simulink model "PEMFuelCellSystem_Cathode_cEGR_ExternalMembraneHumidifier_v01"  (R2025b)
settings: Solver=VariableStepAuto  StartTime=0.0  StopTime=100  MaxStep=0.1  RelTol=1e-3  AbsTol=1e-3
model workspace (MAT data in the model file):
  Gas_properties_block = 'PEMFuelCellSystem_Before_v01/Anode_Hydrogen_BOP/Gas Mixture
Properties'
  Gas_properties_candidates{1} = 'PEMFuelCellSystem_Before_v01/Anode_Hydrogen_BOP/Gas Mixture
    | Properties'
  T_TLU = [223.15 228.15 233.15 238.15 243.15 248.15 253.15 258.15 263.15 268.15 272.66 273.15 273.66 278.15 283.15 288.15 293.15 298.15 303.15 308.15 313.15 318.15 323.15 328.15 333.15 338.15 343.15 348.15 353.15 358.15 363.15 368.15 373.15 378.15 383.15 388.15 393.15 398.15 403.15 408.15 413.15 418.15 423.15 428.15 433.15 438.15 443.15 448.15 453.15 458.15 463.15 468.15 473.15 478.15 483.15 488.15 493.15 498.15 503.15 508.15 513.15 518.15 523.15 528.15 533.15 538.15 543.15 548.15 553.15 558.15 563.15 568.15 573.15 578.15 583.15 588.15 593.15 598.15 603.15 608.15 613.15 618.15 623.15 628.15 633.15 638.15 643.15 646.596 647.596 648.15 653.15 658.15 663.15 668.15 673.15 678.15 683.15 688.15 693.15 698.15 703.15 708.15 713.15 718.15 723.15 728.15 733.15 738.15 743.15 748.15 753.15 758.15 763.15 768.15 773.15]
  air_control_min_current_A = 3.8
  anode_separator_D = 0.02
  anode_separator_T0 = 20
  anode_separator_area = 0.000314159265359
  anode_separator_dp_nominal = 0.0005
  anode_separator_extra_length = 0.04
  anode_separator_laminar_fraction = 0.001
  anode_separator_length = 0.12
  anode_separator_mdot_nominal = 0.01
  anode_separator_p0 = 0.101325
  anode_separator_roughness = 1.5e-05
  anode_tube_D = 0.02
  cathode_channel_dp_nominal_MPa = 0.0368422
  cathode_channel_flow_area_m2 = 0.00403764556423
  cathode_channel_laminar_fraction = 0.5
  cathode_channel_mdot_nominal_kg_s = 0.27182
  cathode_outlet_chamber_V = 0.2
  cathode_separator_D = 0.05
  cathode_separator_T0 = 20
  cathode_separator_area = 0.00407150407905
  cathode_separator_dp_nominal = 0.002
  cathode_separator_extra_length = 0.05
  cathode_separator_laminar_fraction = 0.001
  cathode_separator_length = 0.15
  cathode_separator_mdot_nominal = 0.40798
  cathode_separator_p0 = 0.101325
  cathode_separator_roughness = 1.5e-05
  cathode_tube_D = 0.05
  cegr_comp_map_t_denom_epsilon = 1e-09
  cegr_cond_tau = 1
  cegr_inlet_mixer_p0 = 0.101325
  cegr_outlet_chamber_p0 = 0.101325
  cegr_pipe_D = 0.072
  cegr_pipe_area = 0.00407150407905
  cegr_pipe_extra_length = 0.1
  cegr_pipe_length = 0.5
  cegr_pipe_p0 = 0.101325
  cegr_pipe_roughness = 1.5e-05
  cegr_valve_max_area = 0.001
  cegr_valve_open_min_area = 1e-10
  comp_inlet_mixer_V = 0.1
  comp_mdot_corr_TLU = [0  0.28  0.56; 0  0.26  0.52; 0  0.24  0.48; 0  0.22  0.44; 0  0.2  0.4]
  comp_p_ratio_TLU = [1 1.5 2 2.5 3]
  comp_rpm_TLU = [0 50000 80000]
  coolant_num_layers = 20
  coolant_num_passes = 12
  coolant_tube_D = 0.05
  coolant_w_channels = 1
  drive_cycle_current = [0 0 100 100]
  drive_cycle_power = [0 0 40 40]
  drive_cycle_time = [0 0.5 60.5 600]
  drive_cycle_voltage = [427.6 427.6 410 410]
  env_RH = 0.5
  env_T = 20
  env_p = 0.101325
  env_pSat_H2O = 0.00233931818334
  env_yH20 = 0.0115436377169
  env_yO2 = 0.21
  exhaust_bp_valve_control_Ki_area_per_MPa_s = 0.002
  exhaust_bp_valve_max_area = 0.00134
  exhaust_bp_valve_open_min_area = 1e-10
  focused_anode_boundary_T_C = 20
  focused_anode_feed_p_MPa_abs = 0.3
  focused_anode_inlet_mdot_kg_s = 0.008
  focused_anode_inlet_p_MPa_abs = 0.161325
  focused_anode_outlet_p_MPa_abs = 0.101325
  focused_anode_pipe_area = 0.00246300864041
  focused_anode_pipe_extra_length = 0.1
  focused_anode_pipe_length = 1
  focused_anode_pipe_roughness = 1.5e-05
  focused_anode_yH2 = 0.9997
  focused_cathode_inlet_temperature_C = 58.9
  focused_stack_temperature_C = 80
  humidifier_bypass_mode = "command_gain"
  intercooler_Dh = 0.05
  intercooler_T0 = 20
  intercooler_area = 0.00785398163397
  intercooler_cond_tau = 1
  intercooler_dp_nominal = 0.005
  intercooler_extra_length = 0.05
  intercooler_laminar_fraction = 0.001
  intercooler_length = 0.25
  intercooler_mdot_nominal = 0.40798
  intercooler_p0 = 0.101325
  intercooler_roughness = 1.5e-05
  membrane_humidifier_dry_area_m2 = 0.01
  membrane_humidifier_dry_extra_length_m = 0.1
  membrane_humidifier_dry_hydraulic_diameter_m = 0.05
  membrane_humidifier_dry_length_m = 1
  membrane_humidifier_dry_roughness_m = 1.5e-05
  membrane_humidifier_heat_conductivity_W_per_m_K = 5
  membrane_humidifier_temperature_transfer_time_constant_s = 0.2
  membrane_humidifier_water_transfer_conductance_kg_s_Pa = 1e-08
  membrane_humidifier_water_transfer_time_constant_s = 0.5
  membrane_humidifier_wet_area_m2 = 0.01
  membrane_humidifier_wet_extra_length_m = 0.1
  membrane_humidifier_wet_hydraulic_diameter_m = 0.05
  membrane_humidifier_wet_length_m = 1
  membrane_humidifier_wet_roughness_m = 1.5e-05
  pSat_H2O_TLU = [0.0039376926592 0.00720321689378 0.0128411282011 0.0223441068076 0.0380050105363 0.0632733889962 0.103238678713 0.165273175188 0.259872929049 0.401739659013 0.586936061043 0.611151401419 0.634239116603 0.872575113841 1.22819893069 1.70579291606 2.33931818334 3.16992933887 4.24697083683 5.62901610671 7.38493807375 9.59499884361 12.3519458375 15.7621015462 19.9464343078 25.0415980794 31.2009300265 38.5953958474 47.4144740302 57.866971652 70.1817658151 84.6084663194 101.41799666 120.903091855 143.378712949 169.182379251 198.67442048 232.238151946 270.279976785 313.229419961 361.5390994 415.684640163 476.16453797 543.499978781 618.234621425 700.934350503 792.187006981 892.602104065 1002.81053608 1123.46428821 1255.23615516 1398.81947697 1554.92790047 1724.29517523 1907.67499353 2105.84088402 2319.5861702 2549.72400533 2797.08749693 3062.5299355 3346.92514427 3651.16796903 3976.17493065 4322.88506654 4692.2609923 5085.29022074 5502.98678301 5946.3932056 6416.58290953 6914.66311353 7441.77834442 7999.11468638 8587.90494083 9209.43492415 9865.05121118 10556.1707482 11284.2929275 12051.0149487 12858.0516 13707.2609154 14600.6773719 15540.5540963 16529.415139 17570.1228342 18666.0066449 19821.3641683 21043.5631475 21931.4055737 22037.430306 22037.431306 22037.432306 22037.433306 22037.434306 22037.435306 22037.436306 22037.437306 22037.438306 22037.439306 22037.440306 22037.441306 22037.442306 22037.443306 22037.444306 22037.445306 22037.446306 22037.447306 22037.448306 22037.449306 22037.450306 22037.451306 22037.452306 22037.453306 22037.454306 22037.455306 22037.456306]
  pSat_TLU = [3379.45709837  3379.45809837  3379.45909837  3379.46009837  3379.46109837  3379.46209837  3379.46309837  3379.46409837  3379.46509837  3379.46609837  3379.46709837  3379.46809837  3379.46909837  3379.47009837  3379.47109837  3379.47209837  3379.47309837  3379.47409837  3379.47509837  3379.47609837  3379.47709837  3379.47809837  3379.47909837  3379.48009837  3379.48109837  3379.48209837  3379.48309837  3379.48409837  3379.48509837  3379.48609837  3379.48709837  3379.48809837  3379.48909837  3379.49009837  3379.49109837  3379.49209837  3379.49309837  3379.49409837  3379.49509837  3379.49609837  3379.49709837  3379.49809837  3379.49909837  3379.50009837  3379.50109837  3379.50209837  3379.50309837  3379.50409837  3379.50509837  3379.50609837  3379.50709837  3379.50809837  3379.50909837  3379.51009837  3379.51109837  3379.51209837  3379.51309837  3379.51409837  3379.51509837  3379.51609837  3379.51709837  3379.51809837  3379.51909837  3379.52009837  3379.52109837  3379.52209837  3379.52309837  3379.52409837  3379.52509837  3379.52609837  3379.52709837  3379.52809837  3379.52909837  3379.53009837  3379.53109837  3379.53209837  3379.53309837  3379.53409837  3379.53509837  3379.53609837  3379.53709837  3379.53809837  3379.53909837  3379.54009837  3379.54109837  3379.54209837  3379.54309837  3379.54409837  3379.54509837  3379.54609837  3379.54709837  3379.54809837  3379.54909837  3379.55009837  3379.55109837  3379.55209837  3379.55309837  3379.55409837  3379.55509837  3379.55609837  3379.55709837  3379.55809837  3379.55909837  3379.56009837  3379.56109837  3379.56209837  3379.56309837  3379.56409837  3379.56509837  3379.56609837  3379.56709837  3379.56809837  3379.56909837  3379.57009837  3379.57109837; 5023.40410987  5023.40510987  5023.40610987  5023.40710987  5023.40810987  5023.40910987  5023.41010987  5023.41110987  5023.41210987  5023.41310987  5023.41410987  5023.41510987  5023.41610987  5023.41710987  5023.41810987  5023.41910987  5023.42010987  5023.42110987  5023.42210987  5023.42310987  5023.42410987  5023.42510987  5023.42610987  5023.42710987  5023.42810987  5023.42910987  5023.43010987  5023.43110987  5023.43210987  5023.43310987  5023.43410987  5023.43510987  5023.43610987  5023.43710987  5023.43810987  5023.43910987  5023.44010987  5023.44110987  5023.44210987  5023.44310987  5023.44410987  5023.44510987  5023.44610987  5023.44710987  5023.44810987  5023.44910987  5023.45010987  5023.45110987  5023.45210987  5023.45310987  5023.45410987  5023.45510987  5023.45610987  5023.45710987  5023.45810987  5023.45910987  5023.46010987  5023.46110987  5023.46210987  5023.46310987  5023.46410987  5023.46510987  5023.46610987  5023.46710987  5023.46810987  5023.46910987  5023.47010987  5023.47110987  5023.47210987  5023.47310987  5023.47410987  5023.47510987  5023.47610987  5023.47710987  5023.47810987  5023.47910987  5023.48010987  5023.48110987  5023.48210987  5023.48310987  5023.48410987  5023.48510987  5023.48610987  5023.48710987  5023.48810987  5023.48910987  5023.49010987  5023.49110987  5023.49210987  5023.49310987  5023.49410987  5023.49510987  5023.49610987  5023.49710987  5023.49810987  5023.49910987  5023.50010987  5023.50110987  5023.50210987  5023.50310987  5023.50410987  5023.50510987  5023.50610987  5023.50710987  5023.50810987  5023.50910987  5023.51010987  5023.51110987  5023.51210987  5023.51310987  5023.51410987  5023.51510987  5023.51610987  5023.51710987  5023.51810987; 1277.63968517  1277.64068517  1277.64168517  1277.64268517  1277.64368517  1277.64468517  1277.64568517  1277.64668517  1277.64768517  1277.64868517  1277.64968517  1277.65068517  1277.65168517  1277.65268517  1277.65368517  1277.65468517  1277.65568517  1277.65668517  1277.65768517  1277.65868517  1277.65968517  1277.66068517  1277.66168517  1277.66268517  1277.66368517  1277.66468517  1277.66568517  1277.66668517  1277.66768517  1277.66868517  1277.66968517  1277.67068517  1277.67168517  1277.67268517  1277.67368517  1277.67468517 ...(+2889 chars)]
  radiator_H = 0.5
  radiator_L = 1
  radiator_N_fins = 12000
  radiator_N_tubes = 25
  radiator_W = 0.025
  radiator_air_area_fins = 11.5625
  radiator_air_area_primary = 1.223125
  radiator_cp = 910
  radiator_eta_fin = 0.7
  radiator_fin_spacing = 0.002
  radiator_gap_H = 0.0192708333333
  radiator_rho = 2700
  radiator_t_wall = 0.0001
  radiator_tube_H = 0.0015
  radiator_tube_Leq = 2.5
  routeA_air_control_mode_id = 2
  routeA_air_pid_Ki = 0.5
  routeA_air_pid_Kp = 5
  routeA_anode_inlet_pressure_MPa_abs = 0.161325
  routeA_anode_purge_enable = 1
  routeA_anode_purge_off_n2_mole_fraction = 0.1
  routeA_anode_purge_on_n2_mole_fraction = 0.5
  routeA_anode_recirculation_base_command = 0.2
  routeA_anode_recirculation_current_gain_A_inv = 0.00204081632653
  routeA_anode_rh_setpoint = 1
  routeA_backpressure_control_mode_id = 1
  routeA_cathode_humidifier_gain = 1
  routeA_cathode_rh_setpoint = 1
  routeA_cegr_enabled = 1
  routeA_cegr_valve_mode_id = 1
  routeA_command_profile = [0  0.101325  20  0.21  0.0115436377169  0.045  3  0.5  0.161325  1  1  0  70  20  0.9997  0.161325  1  0.2  0.00204081632653  1  0.5  0.1  80; 0.5  0.101325  20  0.21  0.0115436377169  0.045  3  0.5  0.161325  1  1  0  70  20  0.9997  0.161325  1  0.2  0.00204081632653  1  0.5  0.1  80; 60.5  0.101325  20  0.21  0.0115436377169  0.045  3  0.5  0.161325  1  1  0.1  70  20  0.9997  0.161325  1  0.2  0.00204081632653  1  0.5  0.1  80; 600  0.101325  20  0.21  0.0115436377169  0.045  3  0.5  0.161325  1  1  0.1  70  20  0.9997  0.161325  1  0.2  0.00204081632653  1  0.5  0.1  80]
  routeA_command_profile_baseline = [0.101325 20 0.21 0.0115436377169 0.045 3 0.5 0.1613 1 1 0 70 20 0.9997 0.161325 1 0.2 0.00204081632653 1 0.5 0.1 80]
  routeA_command_profile_fields = ["cathode_source_pressure_MPa_abs" "cathode_source_temperature_C" "cathode_source_o2_mole_fraction" "cathode_source_h2o_mole_fraction" "air_target_mdot_kg_s" "air_target_oer" "air_direct_command" "cathode_outlet_pressure_MPa_abs" "cathode_humidifier_rh" "cathode_humidifier_gain" "cegr_ratio" "anode_source_pressure_MPa_abs" "anode_source_temperature_C" "anode_source_h2_mole_fraction" "anode_inlet_pressure_MPa_abs" "anode_humidifier_rh" "anode_recirculation_base" "anode_recirculation_current_gain_A_inv" "anode_purge_enable" "anode_purge_on_n2_mole_fraction" "anode_purge_off_n2_mole_fraction" "stack_temperature_set_C"]
  routeA_command_profile_schema = "RouteA_Command_Profile_v10"
  routeA_current_default_ref_A = 28
  routeA_egr_control_Ki_area = 3.92699081699e-05
  routeA_egr_control_Kp_area = 0.000196349540849
  routeA_egr_control_mode_id = 1
  routeA_egr_target_input_mode_id = 1
  routeA_egr_valve_actuator_tau = 0.5
  routeA_egr_valve_area_direct = 3.92699081699e-06
  routeA_external_case_enabled = 0
  routeA_parameter_layer = "platform_default"
  routeA_stack_temperature_set_C = 80
  routeA_target_egr_ratio_comp_in = 0.02
  routeA_voltage_current_max_A = 392
  routeA_voltage_current_min_A = 0
  routeA_voltage_default_ref_V = 394.9
  routeA_voltage_pi_Ki = 0.05
  routeA_voltage_pi_Kp = 1
  separator_condensation_enabled = 1
  separator_l2_efficiency = 0.5
  separator_l2_source = "l2_saturation_excess_estimator"
  stack_alpha = 1
  stack_area = 380
  stack_iL = 2.5
  stack_io = 2e-14
  stack_mea_cp = 870
  stack_mea_rho = 1800
  stack_num_cells = 606
  stack_num_channels = 8
  stack_t_gdl = 250
  stack_t_membrane = 125
  stack_w_channels = 1.16496474502
  tank_T = 20
  tank_V = 120
  tank_p = 70
  tank_yH2 = 0.9997
libraries: nesl_utility x57, FuelCell_lib x39, fl_lib x24, slpidlib x4
(part 1 of 6)
settings Model: Creator=ADMIN  LastModifiedBy=ADMIN
settings SolverCC: AutoScaleAbsTol=off  MaxConsecutiveMinStep=10  AlgebraicLoopSolver=TrustRegion  MaxZcPerStep=1.0
settings DataIOCC: SaveFormat=Array  ReturnWorkspaceOutputs=off
settings DebuggingCC: UnconnectedInputMsg=warning  UnconnectedOutputMsg=warning  UnconnectedLineMsg=warning  SymbolicDimsDataTypeCodeGenerationDiagnostic=none
settings ModelReferenceCC: EnableRefExpFcnMdlSchedulingChecks=on
settings SFSimCC: CustomCodeUndefinedFunction=UseInterfaceOnly
settings RTWCC: GPUComputeCapability=3.5  DLArmComputeVersion=19.05
settings SimscapeCC: SimscapeLogType=all  SimscapeLogSimulationStatistics=on  SimscapeLogName=simlog_PEMFuelCellSystem_GasMixture_cEGR_RouteA_v01  SimscapeLogDataHistory=20000.0

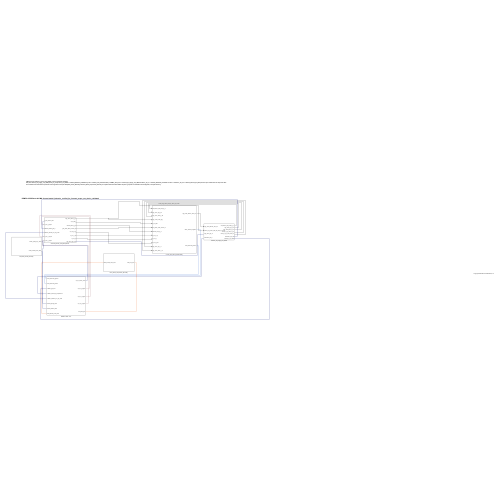
[thumbnail: Simulink's stored preview of the top-level diagram]
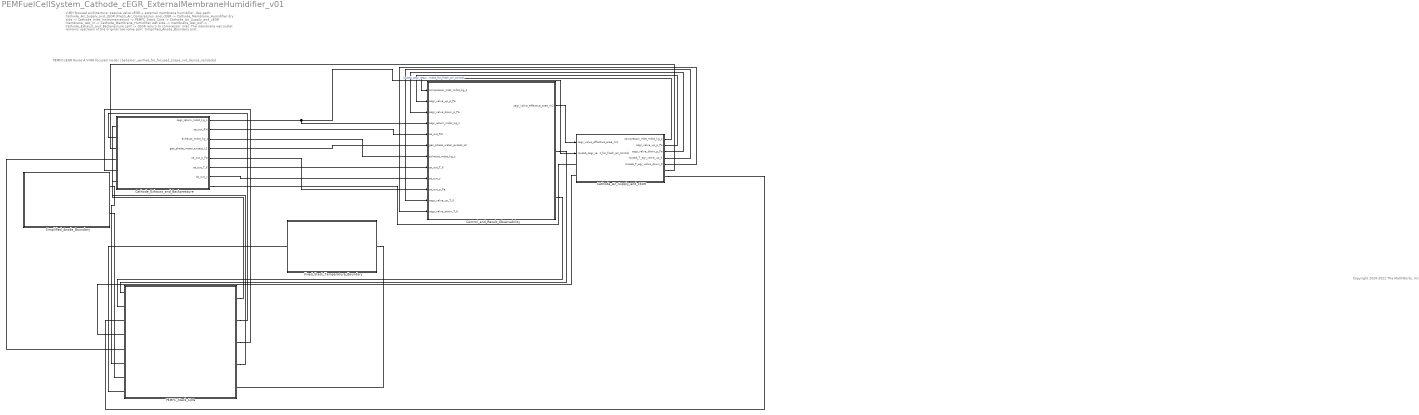
== system PEMFuelCellSystem_Cathode_cEGR_ExternalMembraneHumidifier_v01 ==
  note: PEMFC-cEGR Route A V-MH focused model | behavior_verified_for_focused_scope_not_device_validated
  note: V-MH focused architecture: passive valve cEGR + external membrane humidifier.
      | Gas path: Cathode_Air_Supply_and_cEGR [Fresh_Air_Compression_and_cEGR -> Cathode_Membrane_Humidifier dry side -> Cathode_Inlet_Instrumentation] -> PEMFC_Stack_Core -> Cathode_Air_Supply_and_cEGR membrane_wet_in -> Cathode_Membrane_Humidifier wet side -> membrane_wet_out -> Cathode_Exhaust_and_Backpressure split -> cEGR return to compressor inlet.
      | The membrane wet outlet remains upstream of the original two-valve split. Simplified_Anode_Boundary and Fixed_Stack_Temperature_Boundary are explicit model boundaries. Water output is a gas-phase L2 saturation-excess diagnostic, not liquid inventory.
  note: Copyright 2020-2022 The MathWorks, Inc.
  Cathode_Air_Supply_and_cEGR : Subsystem
  Cathode_Exhaust_and_Backpressure : Subsystem  Description=Common backpressure, gas-phase boundary, return/exhaust split and cathode-outlet result observation.
  Control_and_Result_Observability : Subsystem  Description=Electrical load, cathode/cEGR control, stack measurements and auditable result logging.
  Fixed_Stack_Temperature_Boundary : Subsystem  Description=Fixed stack temperature source and Simscape solver configuration. This is not a cooling-system model.
  PEMFC_Stack_Core : Subsystem  Description=MEA, anode/cathode gas channels, cathode outlet chamber and stack thermal mass.
  Simplified_Anode_Boundary : Subsystem  Description=Hydrogen mass-flow inlet, fixed feed/outlet reservoirs and minimal insulated outlet pipe. No anode humidifier, recirculation or purge BOP.
  wires:
  Cathode_Exhaust_and_Backpressure/6(ca_out_T_K) -> Control_and_Result_Observability/8(ca_out_T_K)
  Cathode_Exhaust_and_Backpressure/5(ca_out_p_Pa) -> Control_and_Result_Observability/10(ca_out_p_Pa)
  Cathode_Exhaust_and_Backpressure/3(exhaust_mdot_kg_s) -> Control_and_Result_Observability/7(exhaust_mdot_kg_s)
  Cathode_Exhaust_and_Backpressure/2(ca_out_RH) -> Control_and_Result_Observability/5(ca_out_RH)
  Cathode_Exhaust_and_Backpressure/1(cegr_return_mdot_kg_s) -> Cathode_Air_Supply_and_cEGR/2(routeA_cegr_return_mdot_for_fresh_air_control), Control_and_Result_Observability/4(cegr_return_mdot_kg_s)  "routeA_cegr_return_mdot_for_fresh_air_control"
  Cathode_Exhaust_and_Backpressure/7(ca_out_y) -> Control_and_Result_Observability/9(ca_out_y)
  Cathode_Exhaust_and_Backpressure/4(gas_phase_water_excess_L2) -> Control_and_Result_Observability/6(gas_phase_water_excess_L2)
  Control_and_Result_Observability/1(cegr_valve_effective_area_m2) -> Cathode_Air_Supply_and_cEGR/1(cegr_valve_effective_area_m2)
  Cathode_Air_Supply_and_cEGR/1(compressor_inlet_mdot_kg_s) -> Control_and_Result_Observability/1(compressor_inlet_mdot_kg_s)
  Cathode_Air_Supply_and_cEGR/2(cegr_valve_up_p_Pa) -> Control_and_Result_Observability/2(cegr_valve_up_p_Pa)
  Cathode_Air_Supply_and_cEGR/3(cegr_valve_down_p_Pa) -> Control_and_Result_Observability/3(cegr_valve_down_p_Pa)
  Cathode_Air_Supply_and_cEGR/4(routeA_T_egr_valve_up_K) -> Control_and_Result_Observability/11(cegr_valve_up_T_K)
  Cathode_Air_Supply_and_cEGR/5(routeA_T_egr_valve_down_K) -> Control_and_Result_Observability/12(cegr_valve_down_T_K)
  connections:
  Control_and_Result_Observability/RConn2 -- PEMFC_Stack_Core/LConn2
  Control_and_Result_Observability/RConn1 -- PEMFC_Stack_Core/LConn1
  Simplified_Anode_Boundary/RConn2 -- PEMFC_Stack_Core/LConn7
  Simplified_Anode_Boundary/RConn1 -- PEMFC_Stack_Core/LConn6
  PEMFC_Stack_Core/RConn2 -- Cathode_Exhaust_and_Backpressure/LConn2
  PEMFC_Stack_Core/RConn4 -- Cathode_Exhaust_and_Backpressure/LConn6
  PEMFC_Stack_Core/LConn5 -- Cathode_Exhaust_and_Backpressure/LConn4
  PEMFC_Stack_Core/RConn1 -- Cathode_Exhaust_and_Backpressure/LConn1
  PEMFC_Stack_Core/RConn3 -- Cathode_Exhaust_and_Backpressure/LConn5
  Fixed_Stack_Temperature_Boundary/LConn1 -- PEMFC_Stack_Core/LConn8
  Fixed_Stack_Temperature_Boundary/RConn1 -- PEMFC_Stack_Core/RConn5
  Cathode_Air_Supply_and_cEGR/RConn1 -- Cathode_Exhaust_and_Backpressure/LConn3
  Cathode_Exhaust_and_Backpressure/RConn1 -- Cathode_Air_Supply_and_cEGR/LConn1
  Cathode_Air_Supply_and_cEGR/RConn2 -- PEMFC_Stack_Core/LConn3
  PEMFC_Stack_Core/LConn4 -- Cathode_Air_Supply_and_cEGR/LConn2

== system PEMFuelCellSystem_Cathode_cEGR_ExternalMembraneHumidifier_v01/Cathode_Air_Supply_and_cEGR ==
  cegr_valve_effective_area_m2 : Inport
  routeA_cegr_return_mdot_for_fresh_air_control : Inport  Port=2
  Cathode_Inlet_Instrumentation : Subsystem  Description=In-line cathode inlet sensors and V-SH RH/species mass-flow recording.
  Cathode_Membrane_Humidifier : Subsystem  Description=V-MH membrane humidifier shell: two official Pipe (FC) gas volumes, equal/opposite H2O MIn/TIn interface, and conservative wall heat transfer. Cross-membrane transfer is added in the next staged step.
  Fresh_Air_Compression_and_cEGR : Subsystem  Description=Function: fresh-air compression/intercooling, compressor-inlet cEGR mixing, passive return valve and insulated return pipe. Input: valve effective area. Outputs: compressor-inlet mass flow plus valve upstream/downstream pressure and temperature. The return-pipe side species source is explicitly zero because V-SH contains no external reaction or separator in this pipe.
  membrane_wet_out : PMIOPort  Side=Right
  cegr_return_gas_in : PMIOPort  Port=2  Side=Left
  cathode_air_to_stack : PMIOPort  Port=3  Side=Right
  membrane_wet_in : PMIOPort  Port=4  Side=Left
  compressor_inlet_mdot_kg_s : Outport
  cegr_valve_up_p_Pa : Outport  Port=2
  cegr_valve_down_p_Pa : Outport  Port=3
  routeA_T_egr_valve_up_K : Outport  Port=4
  routeA_T_egr_valve_down_K : Outport  Port=5
  wires:
  Fresh_Air_Compression_and_cEGR/4(cegr_valve_up_T_K) -> routeA_T_egr_valve_up_K/1  "routeA_T_egr_valve_up_K"
  Fresh_Air_Compression_and_cEGR/2(cegr_valve_up_p_Pa) -> cegr_valve_up_p_Pa/1
  Fresh_Air_Compression_and_cEGR/1(compressor_inlet_mdot_kg_s) -> compressor_inlet_mdot_kg_s/1
  Fresh_Air_Compression_and_cEGR/3(cegr_valve_down_p_Pa) -> cegr_valve_down_p_Pa/1
  Fresh_Air_Compression_and_cEGR/5(cegr_valve_down_T_K) -> routeA_T_egr_valve_down_K/1  "routeA_T_egr_valve_down_K"
  cegr_valve_effective_area_m2/1 -> Fresh_Air_Compression_and_cEGR/1(cegr_valve_effective_area_m2)
  routeA_cegr_return_mdot_for_fresh_air_control/1 -> Fresh_Air_Compression_and_cEGR/2(cegr_return_mdot_kg_s)
  connections:
  Cathode_Membrane_Humidifier/RConn1 -- Cathode_Inlet_Instrumentation/LConn1
  Fresh_Air_Compression_and_cEGR/RConn1 -- Cathode_Membrane_Humidifier/LConn1
  cegr_return_gas_in/RConn1 -- Fresh_Air_Compression_and_cEGR/LConn1
  Cathode_Membrane_Humidifier/RConn2 -- membrane_wet_out/RConn1
  Cathode_Inlet_Instrumentation/RConn1 -- cathode_air_to_stack/RConn1
  membrane_wet_in/RConn1 -- Cathode_Membrane_Humidifier/LConn2

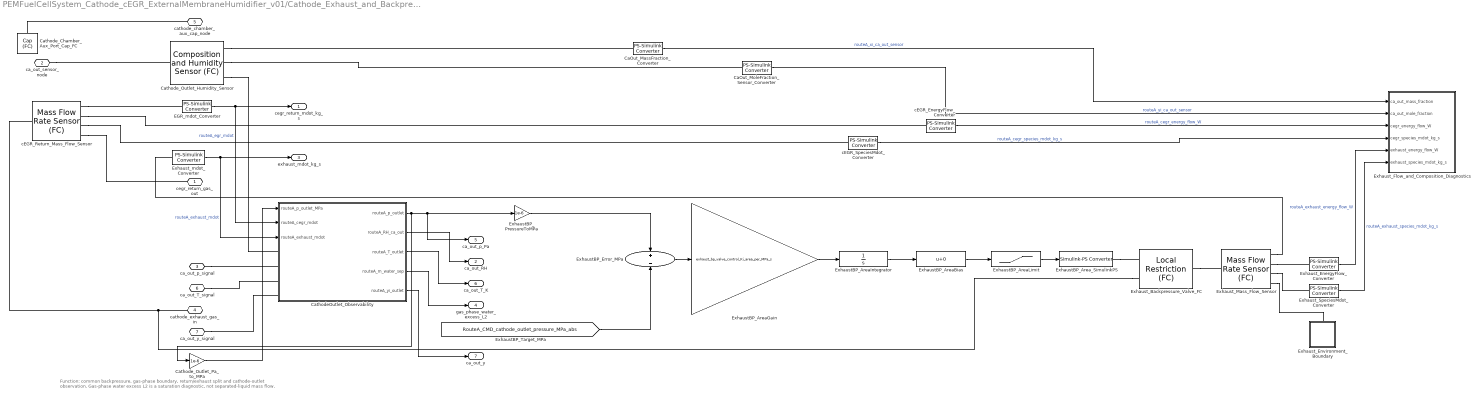
== system PEMFuelCellSystem_Cathode_cEGR_ExternalMembraneHumidifier_v01/Cathode_Exhaust_and_Backpressure ==
  note: Function: common backpressure, gas-phase boundary, return/exhaust split and cathode-outlet observation.
      | Gas-phase water excess L2 is a saturation diagnostic, not separated-liquid mass flow.
  CaOut_MassFraction_Converter : nesl_utility/PS-Simulink Converter  Description=Convert cathode-outlet sensor mass fractions to a named diagnostic signal.  PhysicalDomain=network_engine_domain  SubClassName=ps_output  LeftPortType=input  RightPortType=output  PseudoPeriodic=off  Frequencies=[]  VectorFormat=inherit  Unit=1  AffineConversion=off
  CaOut_MoleFraction_Sensor_Converter : nesl_utility/PS-Simulink Converter  Description=Convert cathode-outlet sensor mole fractions to a named diagnostic signal; this is independent readback of the outlet state.  PhysicalDomain=network_engine_domain  SubClassName=ps_output  LeftPortType=input  RightPortType=output  PseudoPeriodic=off  Frequencies=[]  VectorFormat=inherit  Unit=1  AffineConversion=off
  CathodeOutlet_Observability : Subsystem  Description=Converts cathode-outlet physical signals and branch mass flows into V-SH result observables. Water output is a gas-phase L2 saturation-excess diagnostic, not separated liquid-water inventory.
  Cathode_Chamber_Aux_Port_Cap_FC : FuelCell_lib/elements/Cap (FC)  p_specify=off  p_priority=None  p=101325 Pa  p_nominal_specify=off  p_nominal_value=1  p_nominal_unit=Pa  x_i_specify=off  x_i_priority=None  x_i=[1; 0; 0; 0]  x_i_nominal_specify=off  x_i_nominal_value=1  x_i_nominal_unit=1  T_specify=off  T_priority=None  T=293.15 K  T_nominal_specify=off  T_nominal_value=1  T_nominal_unit=K
      settings: InternalSimscapePortConfiguration="{\"Bottom\":[],\"Left\":[{\"id\":\"A\",\"label\":\"A\",\"type\":\"FuelCell.FuelCell\"}],\"Right\":[],\"Top\":[]}"
  Cathode_Outlet_Humidity_Sensor : FuelCell_lib/sensors/Composition and Humidity Sensor (FC)
      settings: InternalSimscapePortConfiguration="{\"Bottom\":[],\"Left\":[{\"id\":\"A\",\"label\":\"A\",\"type\":\"FuelCell.FuelCell\"}],\"Right\":[{\"id\":\"x_i\",\"label\":\"x_i\",\"type\":\"output\"},{\"id\":\"y_i\",\"label\":\"y_i\",\"type\":\"output\"},{\"id\":\"W\",\"label\":\"W\",\"type\":\"output\"}],\"Top\":[]}"
  Cathode_Outlet_Pa_to_MPa : Gain  Gain=1e-6
  EGR_mdot_Converter : nesl_utility/PS-Simulink Converter  PhysicalDomain=network_engine_domain  SubClassName=ps_output  LeftPortType=input  RightPortType=output  PseudoPeriodic=off  Frequencies=[]  VectorFormat=inherit  Unit=inherit  AffineConversion=off
  ExhaustBP_AreaBias : Bias
  ExhaustBP_AreaGain : Gain  Gain=exhaust_bp_valve_control_Ki_area_per_MPa_s
  ExhaustBP_AreaIntegrator : Integrator  InitialCondition=0.5*exhaust_bp_valve_max_area  LimitOutput=on  UpperSaturationLimit=exhaust_bp_valve_max_area  LowerSaturationLimit=exhaust_bp_valve_open_min_area
  ExhaustBP_AreaLimit : Saturate  UpperLimit=exhaust_bp_valve_max_area  LowerLimit=exhaust_bp_valve_open_min_area
  ExhaustBP_Area_SimulinkPS : nesl_utility/Simulink-PS Converter  PhysicalDomain=network_engine_domain  SubClassName=ps_input  LeftPortType=input  RightPortType=output  PseudoPeriodic=off  Frequencies=[]  NoiseDistribution=none  NoiseParameters=[]  Unit=m^2  AffineConversion=off  FilteringAndDerivatives=provide  SimscapeFilterOrder=1  InputFilterTimeConstant=0.001  UdotUserProvided=0
  ExhaustBP_Error_MPa : Sum  Inputs=+-
  ExhaustBP_PressureToMPa : Gain  Gain=1e-6
  Exhaust_Backpressure_Valve_FC : FuelCell_lib/elements/Local Restriction (FC)  const_area=false  restriction_area=exhaust_bp_valve_open_min_area m^2  min_area=exhaust_bp_valve_open_min_area m^2  max_area=exhaust_bp_valve_max_area m^2  area=0.01 m^2  Cd=0.64  B_lam=0.999
      settings: InternalSimscapePortConfiguration="{\"Bottom\":[],\"Left\":[{\"id\":\"AR\",\"label\":\"AR\",\"type\":\"input\"},{\"id\":\"A\",\"label\":\"A\",\"type\":\"FuelCell.FuelCell\"}],\"Right\":[{\"id\":\"B\",\"label\":\"B\",\"type\":\"FuelCell.FuelCell\"}],\"Top\":[]}"
  Exhaust_EnergyFlow_Converter : nesl_utility/PS-Simulink Converter  Description=Convert exhaust mixture energy flow [W] to a diagnostic signal. Positive direction is sensor A to B.  PhysicalDomain=network_engine_domain  SubClassName=ps_output  LeftPortType=input  RightPortType=output  PseudoPeriodic=off  Frequencies=[]  VectorFormat=inherit  Unit=W  AffineConversion=off
  Exhaust_Environment_Boundary : Subsystem  Tag=PublishSubsystem  Description=Cathode exhaust path to ambient. Applies the exhaust boundary after the common backpressure and gas-phase split.
      settings: PortSchema="{\"entries\":[{\"content\":{\"sides\":[{\"content\":{\"connectorIds\":[]},\"type\":\"ConnectorPlacement.EquallySpacedRectSide\",\"uuid\":\"6344d1cf-22ea-4a51-9588-07afca0fac15\"},{\"content\":{\"connectorIds\":[],\"side\":\"RIGHT\"},\"type\":\"ConnectorPlacement.EquallySpacedRectSide\",\"uuid\":\"a3908f81-9410-4056-87cd-9faba76d3fb8\"},{\"content\":{\"connectorIds\":[\"LConn1\"],\"side\":\"TOP\"},\"type\":\"ConnectorPlacement.EquallySpacedRectSide\",\"uuid\":\"a1c9e24d-adb9-4361-8e9b-feafccbbdb81\"}]},\"type\":\"ConnectorPlacement.EquallySpacedConnector\",\"uuid\":\"d5180d8f-18a0-491d-9fff-909db43c9aea\"}],\"packageUris\":[\"http://schema.mathworks.com/mf0/Connector/R2020b\"],\"version\":\"1.0\"}"
  Exhaust_Flow_and_Composition_Diagnostics : Subsystem  Description=Named observability consumer for cathode-outlet composition and cEGR/exhaust energy and species-flow diagnostics. These signals are measurements only and do not alter the gas network.
  Exhaust_Mass_Flow_Sensor : FuelCell_lib/sensors/Mass Flow Rate Sensor (FC)
      settings: InternalSimscapePortConfiguration="{\"Bottom\":[],\"Left\":[{\"id\":\"A\",\"label\":\"A\",\"type\":\"FuelCell.FuelCell\"}],\"Right\":[{\"id\":\"M\",\"label\":\"M\",\"type\":\"output\"},{\"id\":\"Phi_out\",\"label\":\"Phi\",\"type\":\"output\"},{\"id\":\"M_i\",\"label\":\"M_i\",\"type\":\"output\"},{\"id\":\"B\",\"label\":\"B\",\"type\":\"FuelCell.FuelCell\"}],\"Top\":[]}"
  Exhaust_SpeciesMdot_Converter : nesl_utility/PS-Simulink Converter  Description=Convert exhaust species mass-flow vector [kg/s] to a diagnostic signal. Positive direction is sensor A to B.  PhysicalDomain=network_engine_domain  SubClassName=ps_output  LeftPortType=input  RightPortType=output  PseudoPeriodic=off  Frequencies=[]  VectorFormat=inherit  Unit=kg/s  AffineConversion=off
  Exhaust_mdot_Converter : nesl_utility/PS-Simulink Converter  PhysicalDomain=network_engine_domain  SubClassName=ps_output  LeftPortType=input  RightPortType=output  PseudoPeriodic=off  Frequencies=[]  VectorFormat=inherit  Unit=inherit  AffineConversion=off
  cEGR_EnergyFlow_Converter : nesl_utility/PS-Simulink Converter  Description=Convert cEGR return mixture energy flow [W] to a diagnostic signal. Positive direction is sensor A to B.  PhysicalDomain=network_engine_domain  SubClassName=ps_output  LeftPortType=input  RightPortType=output  PseudoPeriodic=off  Frequencies=[]  VectorFormat=inherit  Unit=W  AffineConversion=off
  cEGR_Return_Mass_Flow_Sensor : FuelCell_lib/sensors/Mass Flow Rate Sensor (FC)
      settings: InternalSimscapePortConfiguration="{\"Bottom\":[],\"Left\":[{\"id\":\"A\",\"label\":\"A\",\"type\":\"FuelCell.FuelCell\"}],\"Right\":[{\"id\":\"M\",\"label\":\"M\",\"type\":\"output\"},{\"id\":\"Phi_out\",\"label\":\"Phi\",\"type\":\"output\"},{\"id\":\"M_i\",\"label\":\"M_i\",\"type\":\"output\"},{\"id\":\"B\",\"label\":\"B\",\"type\":\"FuelCell.FuelCell\"}],\"Top\":[]}"
  cEGR_SpeciesMdot_Converter : nesl_utility/PS-Simulink Converter  Description=Convert cEGR return species mass-flow vector [kg/s] to a diagnostic signal. Positive direction is sensor A to B.  PhysicalDomain=network_engine_domain  SubClassName=ps_output  LeftPortType=input  RightPortType=output  PseudoPeriodic=off  Frequencies=[]  VectorFormat=inherit  Unit=kg/s  AffineConversion=off
  cegr_return_gas_out : PMIOPort  Side=Right
  ca_out_sensor_node : PMIOPort  Port=2  Side=Left
  ca_out_p_signal : PMIOPort  Port=3  Side=Left
  cathode_exhaust_gas_in : PMIOPort  Port=4  Side=Left
  cathode_chamber_aux_cap_node : PMIOPort  Port=5  Side=Left
  ca_out_T_signal : PMIOPort  Port=6  Side=Left
  ca_out_y_signal : PMIOPort  Port=7  Side=Left
  cegr_return_mdot_kg_s : Outport
  ca_out_RH : Outport  Port=2
  exhaust_mdot_kg_s : Outport  Port=3
  gas_phase_water_excess_L2 : Outport  Port=4
  ca_out_p_Pa : Outport  Port=5
  ca_out_T_K : Outport  Port=6
  ca_out_y : Outport  Port=7
  wires:
  ExhaustBP_AreaIntegrator/1 -> ExhaustBP_AreaBias/1
  EGR_mdot_Converter/1 -> cegr_return_mdot_kg_s/1, CathodeOutlet_Observability/2(routeA_cegr_mdot)  "routeA_egr_mdot"
  Exhaust_mdot_Converter/1 -> exhaust_mdot_kg_s/1, CathodeOutlet_Observability/3(routeA_exhaust_mdot)  "routeA_exhaust_mdot"
  cEGR_EnergyFlow_Converter/1 -> Exhaust_Flow_and_Composition_Diagnostics/3(cegr_energy_flow_W)  "routeA_cegr_energy_flow_W"
  Cathode_Outlet_Pa_to_MPa/1 -> CathodeOutlet_Observability/1(routeA_p_outlet_MPa)
  CathodeOutlet_Observability/1(routeA_p_outlet) -> ca_out_p_Pa/1, ExhaustBP_PressureToMPa/1, Cathode_Outlet_Pa_to_MPa/1
  CathodeOutlet_Observability/2(routeA_RH_ca_out) -> ca_out_RH/1
  CaOut_MoleFraction_Sensor_Converter/1 -> Exhaust_Flow_and_Composition_Diagnostics/2(ca_out_mole_fraction)  "routeA_yi_ca_out_sensor"
  CathodeOutlet_Observability/3(routeA_T_outlet) -> ca_out_T_K/1
  CathodeOutlet_Observability/4(routeA_m_water_sep) -> gas_phase_water_excess_L2/1
  CathodeOutlet_Observability/5(routeA_yi_outlet) -> ca_out_y/1
  ExhaustBP_AreaGain/1 -> ExhaustBP_AreaIntegrator/1
  ExhaustBP_PressureToMPa/1 -> ExhaustBP_Error_MPa/1
  [RouteA_CMD_cathode_outlet_pressure_MPa_abs] -> ExhaustBP_Error_MPa/2
  CaOut_MassFraction_Converter/1 -> Exhaust_Flow_and_Composition_Diagnostics/1(ca_out_mass_fraction)  "routeA_xi_ca_out_sensor"
  ExhaustBP_AreaBias/1 -> ExhaustBP_AreaLimit/1
  ExhaustBP_Error_MPa/1 -> ExhaustBP_AreaGain/1
  cEGR_SpeciesMdot_Converter/1 -> Exhaust_Flow_and_Composition_Diagnostics/4(cegr_species_mdot_kg_s)  "routeA_cegr_species_mdot_kg_s"
  ExhaustBP_AreaLimit/1 -> ExhaustBP_Area_SimulinkPS/1
  Exhaust_EnergyFlow_Converter/1 -> Exhaust_Flow_and_Composition_Diagnostics/5(exhaust_energy_flow_W)  "routeA_exhaust_energy_flow_W"
  Exhaust_SpeciesMdot_Converter/1 -> Exhaust_Flow_and_Composition_Diagnostics/6(exhaust_species_mdot_kg_s)  "routeA_exhaust_species_mdot_kg_s"
  connections:
  Exhaust_Mass_Flow_Sensor/RConn3 -- Exhaust_SpeciesMdot_Converter/LConn1
  cEGR_Return_Mass_Flow_Sensor/RConn4 -- cegr_return_gas_out/RConn1
  Exhaust_Mass_Flow_Sensor/RConn1 -- Exhaust_mdot_Converter/LConn1
  cEGR_Return_Mass_Flow_Sensor/RConn2 -- cEGR_EnergyFlow_Converter/LConn1
  Cathode_Chamber_Aux_Port_Cap_FC/LConn1 -- cathode_chamber_aux_cap_node/RConn1
  Exhaust_Mass_Flow_Sensor/RConn2 -- Exhaust_EnergyFlow_Converter/LConn1
  ca_out_T_signal/RConn1 -- CathodeOutlet_Observability/LConn3
  cEGR_Return_Mass_Flow_Sensor/RConn3 -- cEGR_SpeciesMdot_Converter/LConn1
  cEGR_Return_Mass_Flow_Sensor/RConn1 -- EGR_mdot_Converter/LConn1
  ca_out_sensor_node/RConn1 -- Cathode_Outlet_Humidity_Sensor/LConn1
  Cathode_Outlet_Humidity_Sensor/RConn1 -- CaOut_MassFraction_Converter/LConn1
  Cathode_Outlet_Humidity_Sensor/RConn2 -- CaOut_MoleFraction_Sensor_Converter/LConn1
  Cathode_Outlet_Humidity_Sensor/RConn3 -- CathodeOutlet_Observability/LConn1
  ExhaustBP_Area_SimulinkPS/RConn1 -- Exhaust_Backpressure_Valve_FC/LConn1
  ca_out_p_signal/RConn1 -- CathodeOutlet_Observability/LConn2
  Exhaust_Mass_Flow_Sensor/RConn4 -- Exhaust_Environment_Boundary/LConn1
  ca_out_y_signal/RConn1 -- CathodeOutlet_Observability/LConn4
  Exhaust_Backpressure_Valve_FC/RConn1 -- Exhaust_Mass_Flow_Sensor/LConn1
  Exhaust_Backpressure_Valve_FC/LConn2 -- cathode_exhaust_gas_in/RConn1 -- cEGR_Return_Mass_Flow_Sensor/LConn1

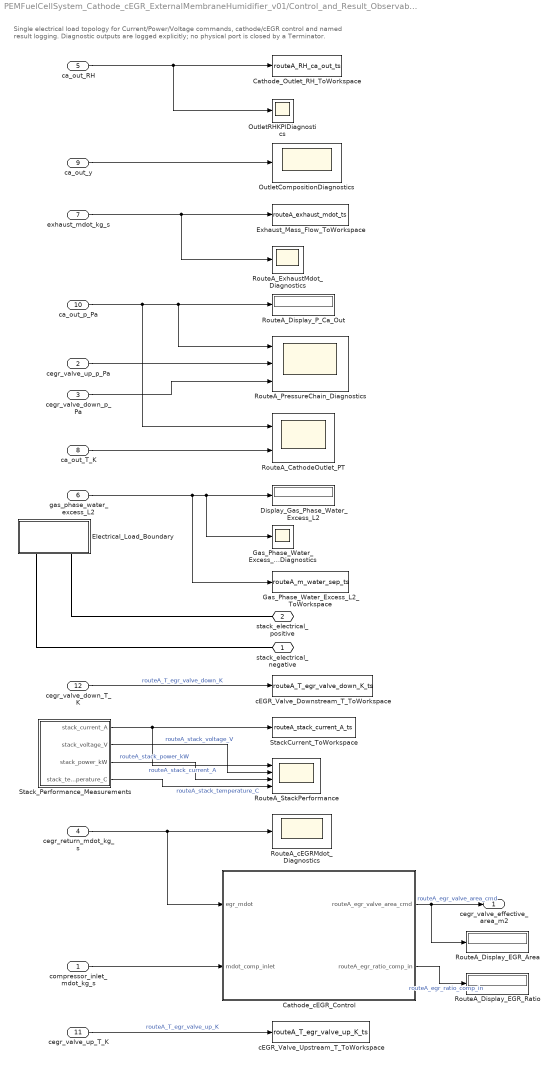
== system PEMFuelCellSystem_Cathode_cEGR_ExternalMembraneHumidifier_v01/Control_and_Result_Observability ==
  note: Single electrical load topology for Current/Power/Voltage commands, cathode/cEGR control and named result logging.
      | Diagnostic outputs are logged explicitly; no physical port is closed by a Terminator.
  compressor_inlet_mdot_kg_s : Inport
  cegr_valve_up_p_Pa : Inport  Port=2
  cegr_valve_down_p_Pa : Inport  Port=3
  cegr_return_mdot_kg_s : Inport  Port=4
  ca_out_RH : Inport  Port=5
  gas_phase_water_excess_L2 : Inport  Port=6
  exhaust_mdot_kg_s : Inport  Port=7
  ca_out_T_K : Inport  Port=8
  ca_out_y : Inport  Port=9
  ca_out_p_Pa : Inport  Port=10
  cegr_valve_up_T_K : Inport  Description=Valve-upstream gas temperature [K], from the cEGR supply/return subsystem.  Port=11
  cegr_valve_down_T_K : Inport  Description=Valve-downstream gas temperature [K], from the cEGR supply/return subsystem.  Port=12
  Cathode_Outlet_RH_ToWorkspace : ToWorkspace  VariableName=routeA_RH_ca_out_ts  SaveFormat=Structure With Time
  Cathode_cEGR_Control : Subsystem  Description=Computes fresh-air and passive cEGR valve commands from compressor-inlet and return-flow measurements.
  Display_Gas_Phase_Water_Excess_L2 : Display
  Electrical_Load_Boundary : Subsystem  Tag=PublishSubsystem  Description=Applies Current, Power or Voltage command through the single stack electrical load path.  mask(Electrical Load){input_type=Voltage}
      mask prompts: input_type "Select one of the following scenarios:"
      mask help: Electrical boundary mode selector. input_type activates one demand variant inside Inputs: Current (I_cmd direct), Power (P_cmd -> I_cmd), or Voltage (V_cmd -> PI -> I_cmd). One mode per run; set per-case via SimulationInput.setBlockParameter(...,'input_type',...).
      settings: PortSchema="{\"entries\":[{\"content\":{\"sides\":[{\"content\":{\"connectorIds\":[]},\"type\":\"ConnectorPlacement.EquallySpacedRectSide\",\"uuid\":\"cf26c57a-4aaa-4eca-a1cf-dab3379228b7\"},{\"content\":{\"connectorIds\":[],\"side\":\"RIGHT\"},\"type\":\"ConnectorPlacement.EquallySpacedRectSide\",\"uuid\":\"bd4a28c6-f8d3-4492-9f61-a12eb17ccdd3\"},{\"content\":{\"connectorIds\":[],\"side\":\"TOP\"},\"type\":\"ConnectorPlacement.EquallySpacedRectSide\",\"uuid\":\"7f54a4db-ccf4-4e3a-a135-4ada067d241f\"},{\"content\":{\"connectorIds\":[\"RConn1\",\"RConn2\"],\"side\":\"BOTTOM\"},\"type\":\"ConnectorPlacement.EquallySpacedRectSide\",\"uuid\":\"8817983d-3f79-43b3-9594-6d12f7dcf066\"}]},\"type\":\"ConnectorPlacement.EquallySpacedConnector\",\"uuid\":\"79253ea6-cd7f-4983-840a-f5cee3a4dd91\"}],\"packageUris\":[\"http://schema.mathworks.com/mf0/Connector/R2020b\"],\"version\":\"1.0\"}"
      mask TypeOptions input_type: Current | Power | Voltage
      mask Callback input_type:
      | activeVariant = get_param(gcb, 'input_type');
      | set_param([gcb '/Inputs'], 'OverrideUsingVariant', activeVariant)
      mask Display:
      | blk = get_param([gcb, '/Inputs'], 'CompiledActiveChoiceBlock');
      | eval(get_param(blk, 'MaskDisplay'))
  Exhaust_Mass_Flow_ToWorkspace : ToWorkspace  VariableName=routeA_exhaust_mdot_ts  SaveFormat=Structure With Time  SampleTime=-1
  Gas_Phase_Water_Excess_L2_Diagnostics : Scope
  Gas_Phase_Water_Excess_L2_ToWorkspace : ToWorkspace  VariableName=routeA_m_water_sep_ts  SaveFormat=Structure With Time
      settings: Description=Legacy workspace variable routeA_m_water_sep_ts stores the L2 gas-phase saturation-excess diagnostic; it is not separated-liquid mass flow.
  OutletCompositionDiagnostics : Scope
  OutletRHKPIDiagnostics : Scope
  RouteA_CathodeOutlet_PT : Scope  NumInputPorts=2
  RouteA_Display_EGR_Area : Display
  RouteA_Display_EGR_Ratio : Display
  RouteA_Display_P_Ca_Out : Display
  RouteA_ExhaustMdot_Diagnostics : Scope
  RouteA_PressureChain_Diagnostics : Scope  NumInputPorts=3
  RouteA_StackPerformance : Scope  NumInputPorts=4
      settings: Title=Current (A)  ActiveDisplayYMinimum=-30.6721  ActiveDisplayYMaximum=276.0489
  RouteA_cEGRMdot_Diagnostics : Scope
  StackCurrent_ToWorkspace : ToWorkspace  VariableName=routeA_stack_current_A_ts  SaveFormat=Structure With Time
  Stack_Performance_Measurements : Subsystem  Description=Converts stack electrical and thermal physical signals into named I, V, P and temperature observables.
  cEGR_Valve_Downstream_T_ToWorkspace : ToWorkspace  VariableName=routeA_T_egr_valve_down_K_ts  SaveFormat=Structure With Time
      settings: Description=Log the measured valve-downstream gas temperature [K] for cEGR thermal/condensation diagnostics.
  cEGR_Valve_Upstream_T_ToWorkspace : ToWorkspace  VariableName=routeA_T_egr_valve_up_K_ts  SaveFormat=Structure With Time
      settings: Description=Log the measured valve-upstream gas temperature [K] for cEGR thermal/condensation diagnostics.
  stack_electrical_negative : PMIOPort  Side=Right
  stack_electrical_positive : PMIOPort  Port=2  Side=Right
  cegr_valve_effective_area_m2 : Outport
  wires:
  cegr_valve_down_p_Pa/1 -> RouteA_PressureChain_Diagnostics/3
  cegr_valve_up_p_Pa/1 -> RouteA_PressureChain_Diagnostics/2
  exhaust_mdot_kg_s/1 -> Exhaust_Mass_Flow_ToWorkspace/1, RouteA_ExhaustMdot_Diagnostics/1
  ca_out_RH/1 -> Cathode_Outlet_RH_ToWorkspace/1, OutletRHKPIDiagnostics/1
  ca_out_p_Pa/1 -> RouteA_PressureChain_Diagnostics/1, RouteA_Display_P_Ca_Out/1, RouteA_CathodeOutlet_PT/1
  ca_out_y/1 -> OutletCompositionDiagnostics/1
  ca_out_T_K/1 -> RouteA_CathodeOutlet_PT/2
  gas_phase_water_excess_L2/1 -> Gas_Phase_Water_Excess_L2_Diagnostics/1, Display_Gas_Phase_Water_Excess_L2/1, Gas_Phase_Water_Excess_L2_ToWorkspace/1
  cegr_valve_down_T_K/1 -> cEGR_Valve_Downstream_T_ToWorkspace/1  "routeA_T_egr_valve_down_K"
  Stack_Performance_Measurements/1(stack_current_A) -> StackCurrent_ToWorkspace/1, RouteA_StackPerformance/1  "routeA_stack_current_A"
  Stack_Performance_Measurements/2(stack_voltage_V) -> RouteA_StackPerformance/2  "routeA_stack_voltage_V"
  Stack_Performance_Measurements/3(stack_power_kW) -> RouteA_StackPerformance/3  "routeA_stack_power_kW"
  Stack_Performance_Measurements/4(stack_temperature_C) -> RouteA_StackPerformance/4  "routeA_stack_temperature_C"
  cegr_return_mdot_kg_s/1 -> Cathode_cEGR_Control/1(egr_mdot), RouteA_cEGRMdot_Diagnostics/1
  compressor_inlet_mdot_kg_s/1 -> Cathode_cEGR_Control/2(mdot_comp_inlet)
  cegr_valve_up_T_K/1 -> cEGR_Valve_Upstream_T_ToWorkspace/1  "routeA_T_egr_valve_up_K"
  Cathode_cEGR_Control/1(routeA_egr_valve_area_cmd) -> cegr_valve_effective_area_m2/1, RouteA_Display_EGR_Area/1  "routeA_egr_valve_area_cmd"
  Cathode_cEGR_Control/2(routeA_egr_ratio_comp_in) -> RouteA_Display_EGR_Ratio/1  "routeA_egr_ratio_comp_in"
  connections:
  Electrical_Load_Boundary/RConn2 -- stack_electrical_positive/RConn1
  Electrical_Load_Boundary/RConn1 -- stack_electrical_negative/RConn1

== system PEMFuelCellSystem_Cathode_cEGR_ExternalMembraneHumidifier_v01/Fixed_Stack_Temperature_Boundary ==
  note: Fixed stack-temperature boundary using focused_stack_temperature_C plus the Simscape solver configuration.
      | This subsystem is not a cooling-loop or thermal-management BOP model.
  Simscape_Solver_Configuration : nesl_utility/Solver Configuration  PhysicalDomain=network_engine_domain  SubClassName=solver  LeftPortType=input  RightPortType=generic  Tones=[]  Harmonics=[]  SimulateNoise=off  Profile=off  UseLocalSampling=off  EnableSwitchedLinearOptims=on  FrequencyDomain=off  UseCCode=off  RelTol=0.001  AbsTol=1e-06  MinStep=1e-09  ToWorkspace=off  RevertToSquareIcSolve=off  NumHomotopyIterations=100  PhasorMode=off  PhasorModeNumHarmonics=1  ConsistencySolver=NEWTON_XTOL_AFTER_FTOL  IndexReductionMethod=DerivativeReplacement  DoDC=off  ResidualTolerance=1e-09  ConsistencyTolSource=GLOBAL  ConsistencyAbsTol=0.001  ConsistencyRelTol=0.001  ConsistencyTolFactor=0.001  UseLocalSolver=off  LocalSolverChoice=NE_BACKWARD_EULER_ADVANCER  ResolveIndetEquations=on  FunctionEvalNumThread=1  LocalSolverSampleTime=0.001  DoFixedCost=off  MaxNonlinIter=3  MaxModeIter=2  ComputeImpulses=off  ImpulseIterations=2  LinearAlgebra=auto  LinearAlgebraNumThread=0  EquationFormulation=NE_TIME_EF  DelaysMemoryBudget=1024  AutomaticFiltering=on  FilteringTimeConstant=0.001  PartitionStorageMethod=AS_NEEDED  PartitionMemoryBudget=1024  PartitionMethod=ROBUST  MultibodyUseLocalSolver=off  MultibodyLocalSolverChoice=ODE1  MultibodyLocalSolverSampleTime=0.001
  Stack_Fixed_Temperature_Source : fl_lib/Thermal/Thermal Sources/Temperature Source  Description=Imposes focused_stack_temperature_C on the simplified V-SH stack thermal boundary.  temperature=focused_stack_temperature_C degC
  stack_thermal_mass_node : PMIOPort  Side=Left
  mea_heat_port : PMIOPort  Port=2  Side=Right
  connections:
  mea_heat_port/RConn1 -- Simscape_Solver_Configuration/RConn1 -- Stack_Fixed_Temperature_Source/LConn1 -- stack_thermal_mass_node/RConn1
